simulink model "DC1_MSA"  (Simulink 7.9)
settings: Solver=ode45  StartTime=0.0  StopTime=time_span  RelTol=1e-3
undefined symbols (not defined in the file): noise_on, outstr, p, samp_time
libraries: simulink x1
settings Model: Creator=Jim  LastModifiedBy=danai
settings DataIOCC: LimitDataPoints=off  SaveTime=off  TimeSaveName=t
settings OptimizationCC: InitFltsAndDblsToZero=on
settings DebuggingCC: SaveWithParameterizedLinksMsg=none  FcnCallInpInsideContextMsg=Use local settings  StrictBusMsg=Warning
settings GRTTargetCC: TargetFcnLib=ansi_tfl_tmw.mat  CombineOutputUpdateFcns=off  GRTInterface=on

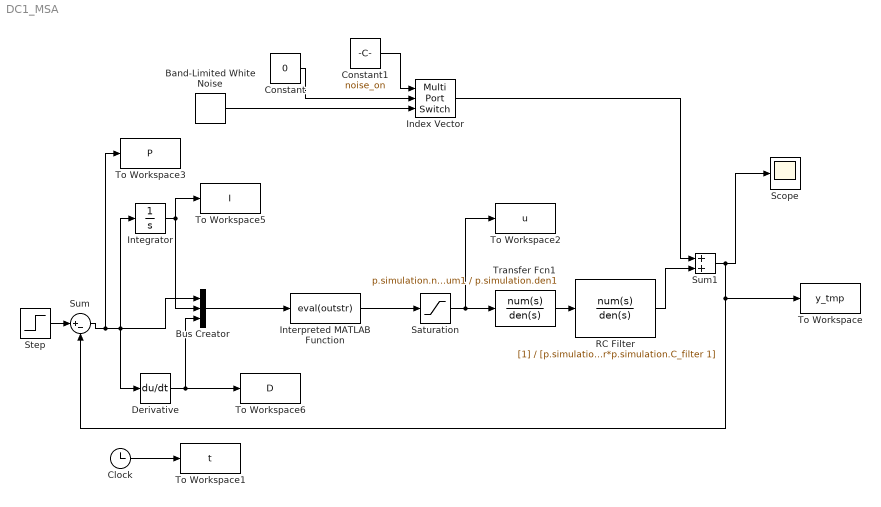
== system DC1_MSA ==
  Band-Limited White Noise : simulink/Sources/Band-Limited White Noise  Cov=[0.0001]  Ts=0.1  seed=[23341]
  Bus Creator : BusCreator  Inputs=3
  Clock : Clock
  Constant : Constant  Value=0
  Constant1 : Constant  Value=noise_on
  Derivative : Derivative
  Index Vector : MultiPortSwitch  DataPortOrder=Zero-based contiguous  Inputs=2  zeroidx=on
  Integrator : Integrator
  Interpreted MATLAB Function : MATLABFcn  MATLABFcn=eval(outstr)
  RC Filter : TransferFcn  Denominator=[p.simulation.R_filter*p.simulation.C_filter 1]
  Saturation : Saturate  UpperLimit=10  LowerLimit=-10  LinearizeAsGain=off  ZeroCross=off
  Scope : Scope
  Step : Step  Time=0  After=p.simulation.Vref  SampleTime=0
  Sum : Sum  Inputs=|+-
  Sum1 : Sum  Inputs=|++
  To Workspace : ToWorkspace  VariableName=y_tmp  SampleTime=samp_time
  To Workspace1 : ToWorkspace  VariableName=t  SampleTime=samp_time
  To Workspace2 : ToWorkspace  VariableName=u  SampleTime=samp_time
  To Workspace3 : ToWorkspace  VariableName=P  SampleTime=samp_time
  To Workspace5 : ToWorkspace  VariableName=I  SampleTime=samp_time
  To Workspace6 : ToWorkspace  VariableName=D  SampleTime=samp_time
  Transfer Fcn1 : TransferFcn  Numerator=p.simulation.num1  Denominator=p.simulation.den1
  wires:
  Clock/1 -> To Workspace1/1
  RC Filter/1 -> Sum1/2
  Constant1/1 -> Index Vector/1
  Constant/1 -> Index Vector/2
  Band-Limited White Noise/1 -> Index Vector/3
  Index Vector/1 -> Sum1/1
  Sum/1 -> Integrator/1, Derivative/1, Bus Creator/1, To Workspace3/1
  Step/1 -> Sum/1
  Sum1/1 -> Scope/1, To Workspace/1, Sum/2
  Derivative/1 -> Bus Creator/3, To Workspace6/1
  Integrator/1 -> To Workspace5/1, Bus Creator/2
  Bus Creator/1 -> Interpreted MATLAB Function/1
  Interpreted MATLAB Function/1 -> Saturation/1
  Saturation/1 -> Transfer Fcn1/1, To Workspace2/1
  Transfer Fcn1/1 -> RC Filter/1
